simulink model "Simulink_PID"  (R2020a)
settings: Solver=VariableStepAuto  StartTime=0.0  StopTime=1000  RelTol=1e-3
libraries: dspsrcs4 x1
settings Model: Creator=Laura  LastModifiedBy=juan
settings SFSimCC: CustomCodeUndefinedFunction=UseInterfaceOnly

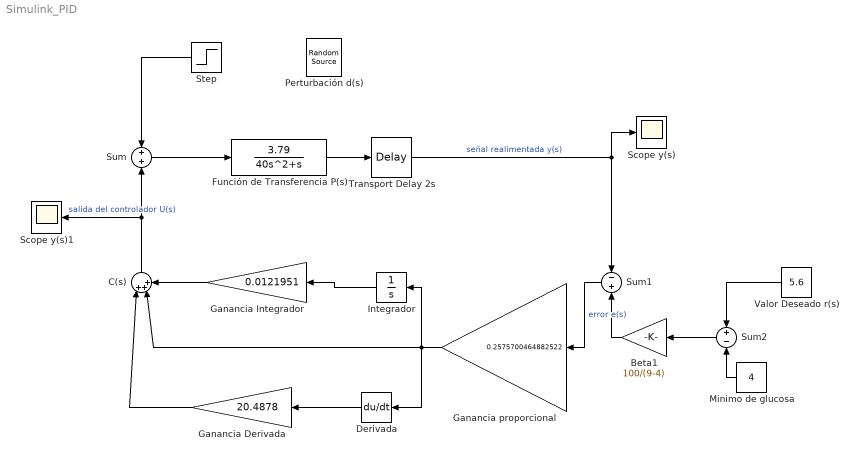
== system Simulink_PID ==
  " C(s)" : Sum  Inputs=|+++
  Beta1 : Gain  Gain=100/(9-4)
  Derivada : Derivative
  Función de Transferencia P(s) : TransferFcn  Numerator=[3.79]  Denominator=[40 1 0]
  Ganancia Derivada : Gain  Gain=20.4878
  Ganancia Integrador : Gain  Gain=0.0121951
  Ganancia proporcional : Gain  Gain=0.2575700464882522
  Integrador : Integrator
  Minimo de glucosa : Constant  Value=4
  "Perturbación d(s) " : dspsrcs4/Random Source  SrcType=Uniform  NormMethod=Ziggurat  CltLength=12  MinVal=0  MaxVal=1  MeanVal=0  VarVal=1  RepMode=Not repeatable  rawSeed=1  IsInherit=off  SampMode=Discrete  SampTime=1  SampFrame=1  DataType=Double  OutComplex=Real  OutputFrames=off
  Scope y(s) : Scope
  Scope y(s)1 : Scope
  Step : Step  Time=200  After=20  SampleTime=0
  Sum : Sum
  Sum1 : Sum  Inputs=-+
  Sum2 : Sum  Inputs=+-
  Transport Delay 2s : TransportDelay  DelayTime=2
  Valor Deseado r(s) : Constant  Value=5.6
  wires:
  Integrador/1 -> Ganancia Integrador/1
  Derivada/1 -> Ganancia Derivada/1
  Ganancia Integrador/1 -> " C(s)"/3
  Ganancia proporcional/1 -> Derivada/1, " C(s)"/2, Integrador/1
  Ganancia Derivada/1 -> " C(s)"/1
  " C(s)"/1 -> Scope y(s)1/1, Sum/2  "salida del controlador U(s)"
  Sum/1 -> Función de Transferencia P(s)/1
  Transport Delay 2s/1 -> Scope y(s)/1, Sum1/1  "señal realimentada y(s)"
  Función de Transferencia P(s)/1 -> Transport Delay 2s/1
  Sum1/1 -> Ganancia proporcional/1  "error e(s)"
  Sum2/1 -> Beta1/1
  Minimo de glucosa/1 -> Sum2/2
  Valor Deseado r(s)/1 -> Sum2/1
  Beta1/1 -> Sum1/2
  Step/1 -> Sum/1
